simulink model "LugL6sStEnCtrl"  (R2018b)
settings: Solver=FixedStepDiscrete  StartTime=0.0  StopTime=10.0  FixedStep=0.01  RelTol=1e-3
undefined symbols (not defined in the file or in its folder): data, ThdRwLtStBkReclnEn_Clear, ThdRwLtStBkReclnEn_Set, ThdRwLtStFwdBkwdEn_Clear, ThdRwLtStFwdBkwdEn_Set
libraries: simulink x1
settings Model: Creator=sn2xws  LastModifiedBy=sn2xws
settings Model: ModifiedHistory=|
  | 2024.6.19 V1.0.0 557 模式流程
  | 2024.8.15 lug模式靠背一起动
settings DataIOCC: SaveFormat=StructureWithTime
settings OptimizationCC: DefaultParameterBehavior=Inlined  EnhancedBackFolding=on  PassReuseOutputArgsAs=Individual arguments  ZeroExternalMemoryAtStartup=off  ZeroInternalMemoryAtStartup=off  OptimizeBlockOrder=speed  DifferentSizesBufferReuse=on  OptimizationCustomize=off
settings DebuggingCC: ParameterTunabilityLossMsg=error
settings SFSimCC: MATLABDynamicMemAlloc=off
settings RTWCC: SystemTargetFile=autosar.tlc  GenCodeOnly=on  TemplateMakefile=ert_default_tmf  Description=AUTOSAR  GenerateReport=on  IncludeHyperlinkInReport=on  LaunchReport=on  GenerateTraceInfo=on  GenerateTraceReport=on  GenerateTraceReportSl=on  GenerateTraceReportSf=on  GenerateTraceReportEml=on
settings CodeAppCC: ForceParamTrailComments=on  IgnoreCustomStorageClasses=off  OperatorAnnotations=on  SimulinkDataObjDesc=on  SFDataObjDesc=on  InsertBlockDesc=on
settings STFCustomTargetCC: TargetLangStandard=C99 (ISO)  MultiwordLength=256  ParMdlRefBuildCompliant=on  CompOptLevelCompliant=on  IncludeMdlTerminateFcn=off  CombineOutputUpdateFcns=on  SuppressErrorStatus=on  ERTCustomFileBanners=on  SupportNonFinite=off  SupportComplex=off  SupportContinuousTime=off  SupportNonInlinedSFcns=off  RemoveResetFunc=on  MATLABClassNameForMDSCustomization=Simulink.SoftwareTarget.ERTCustomization  AutosarCompliant=on  UseToolchainInfoCompliant=on  LookupTableObjectStructAxisOrder=2,1,3,4,...  LUTObjectStructOrderEvenSpacing=Size,Table,Breakpoints  SystemTargetFile=autosar.tlc
settings ERTTargetCC: TargetLangStandard=C99 (ISO)  ConcurrentExecutionCompliant=off  IncludeMdlTerminateFcn=off  SuppressErrorStatus=on  SupportNonFinite=off  SupportComplex=off  ModelStepFunctionPrototypeControlCompliant=off  CPPClassGenCompliant=off  AutosarCompliant=on  LookupTableObjectStructAxisOrder=2,1,3,4,...  LUTObjectStructOrderEvenSpacing=Size,Table,Breakpoints  InlinedParameterPlacement=NonHierarchical  ERTCustomFileTemplate=example_file_process.tlc  ERTFilePackagingFormat=Compact

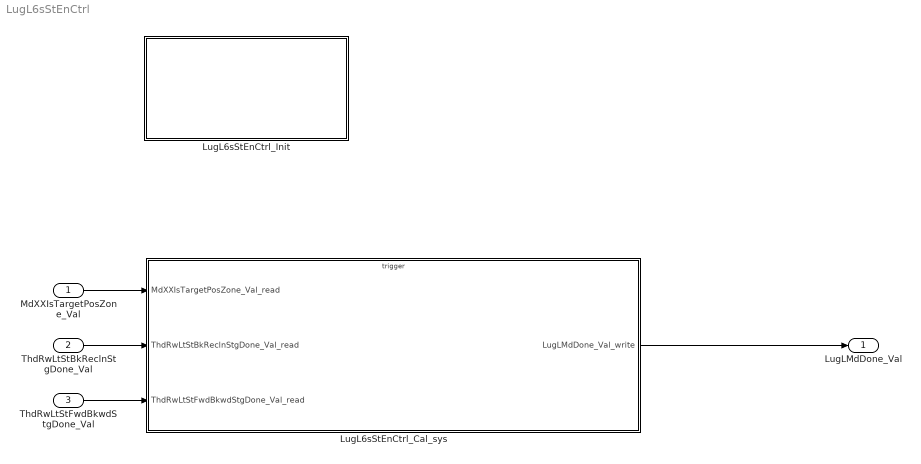
== system LugL6sStEnCtrl ==
  MdXXIsTargetPosZone_Val : Inport  OutDataTypeStr=uint32  PortDimensions=1
  ThdRwLtStBkReclnStgDone_Val : Inport  Port=2  OutDataTypeStr=boolean  PortDimensions=1
  ThdRwLtStFwdBkwdStgDone_Val : Inport  Port=3  OutDataTypeStr=boolean  PortDimensions=1
  LugL6sStEnCtrl_Cal_sys : Subsystem
  LugL6sStEnCtrl_Init : Subsystem
  LugLMdDone_Val : Outport  OutDataTypeStr=uint8  PortDimensions=1
  wires:
  MdXXIsTargetPosZone_Val/1 -> LugL6sStEnCtrl_Cal_sys/1(MdXXIsTargetPosZone_Val_read)
  ThdRwLtStBkReclnStgDone_Val/1 -> LugL6sStEnCtrl_Cal_sys/2(ThdRwLtStBkReclnStgDone_Val_read)
  ThdRwLtStFwdBkwdStgDone_Val/1 -> LugL6sStEnCtrl_Cal_sys/3(ThdRwLtStFwdBkwdStgDone_Val_read)
  LugL6sStEnCtrl_Cal_sys/1(LugLMdDone_Val_write) -> LugLMdDone_Val/1

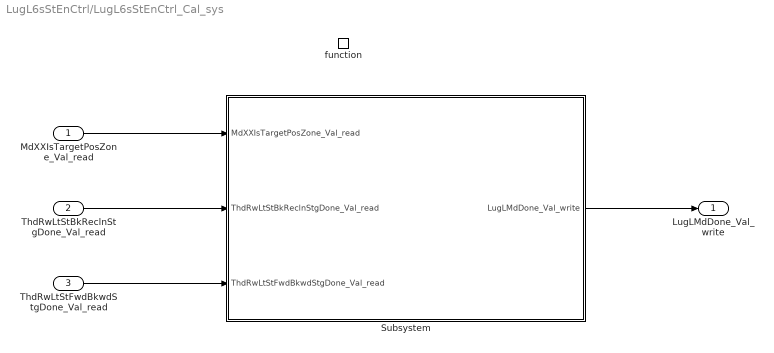
== system LugL6sStEnCtrl/LugL6sStEnCtrl_Cal_sys ==
  MdXXIsTargetPosZone_Val_read : Inport
  ThdRwLtStBkReclnStgDone_Val_read : Inport  Port=2
  ThdRwLtStFwdBkwdStgDone_Val_read : Inport  Port=3
  function : TriggerPort  TriggerType=function-call  IsSimulinkFunction=on  FunctionName=LugL6sStEnCtrl_Cal  VariantControl=(inherit)
  Subsystem : Subsystem
  LugLMdDone_Val_write : Outport
      settings: EnsureOutportIsVirtual=on
  wires:
  MdXXIsTargetPosZone_Val_read/1 -> Subsystem/1(MdXXIsTargetPosZone_Val_read)
  ThdRwLtStBkReclnStgDone_Val_read/1 -> Subsystem/2(ThdRwLtStBkReclnStgDone_Val_read)
  ThdRwLtStFwdBkwdStgDone_Val_read/1 -> Subsystem/3(ThdRwLtStFwdBkwdStgDone_Val_read)
  Subsystem/1(LugLMdDone_Val_write) -> LugLMdDone_Val_write/1

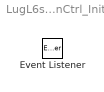
== system LugL6sStEnCtrl/LugL6sStEnCtrl_Init ==
  Event Listener : EventListener  EventName=reset

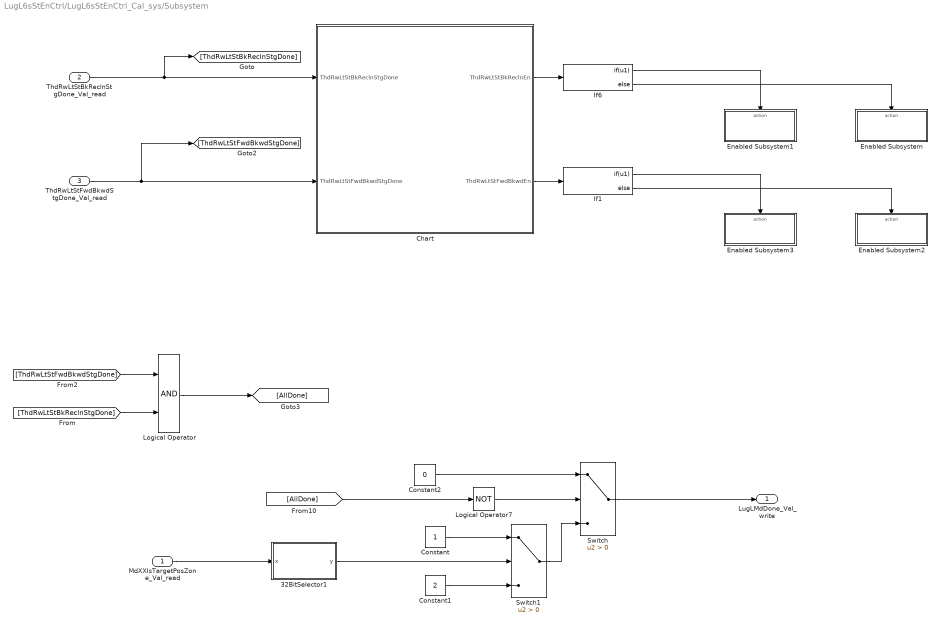
== system LugL6sStEnCtrl/LugL6sStEnCtrl_Cal_sys/Subsystem ==
  MdXXIsTargetPosZone_Val_read : Inport
  ThdRwLtStBkReclnStgDone_Val_read : Inport  Port=2
  ThdRwLtStFwdBkwdStgDone_Val_read : Inport  Port=3
  32BitSelector1 : Subsystem  mask(32 Bit Selector){BitNum=7}
      mask prompts: BitNum "Select Bit Number"
      mask help: Allows selection of a particular bit (0-31) out of a packed word up to 32 bits long. Output will be true if the bit number selected via the mask parameter is equal to one.
      mask TypeOptions BitNum: 0 | 1 | 2 | 3 | 4 | 5 | 6 | 7 | 8 | 9 | 10 | 11 | 12 | 13 | 14 | 15 | 16 | 17 | 18 | 19 | 20 | 21 | 22 | 23 | 24 | 25 | 26 | 27 | 28 | 29 | 30 | 31
      mask Display:
      | text(0.5, 0.8,'BIT','horizontalAlignment','center')
      | text(0.5, 0.5,'SELECTOR','horizontalAlignment','center')
      | text(0.5, 0.2,['-- Bit ',char(get_param(gcb,'BitNum')),' --'],'horizontalAlignment','center')
  Chart : Stateflow chart  TreatAsAtomicUnit=on
  Constant : Constant  OutDataTypeStr=uint8
  Constant1 : Constant  Value=2  OutDataTypeStr=uint8
  Constant2 : Constant  Value=0  OutDataTypeStr=uint8
  Enabled Subsystem : Subsystem  TreatAsAtomicUnit=on
  Enabled Subsystem1 : Subsystem  TreatAsAtomicUnit=on
  Enabled Subsystem2 : Subsystem  TreatAsAtomicUnit=on
  Enabled Subsystem3 : Subsystem  TreatAsAtomicUnit=on
  If1 : If  IfExpression=u1
  If6 : If  IfExpression=u1
  Logical Operator : Logic  AllPortsSameDT=off  OutDataTypeStr=boolean
  Logical Operator7 : Logic  Operator=NOT  AllPortsSameDT=off  OutDataTypeStr=boolean
  Switch : Switch  Criteria=u2 > Threshold
  Switch1 : Switch  Criteria=u2 > Threshold
  LugLMdDone_Val_write : Outport
      settings: EnsureOutportIsVirtual=on
  wires:
  Switch/1 -> LugLMdDone_Val_write/1
  Constant1/1 -> Switch1/3
  MdXXIsTargetPosZone_Val_read/1 -> 32BitSelector1/1(x)
  Switch1/1 -> Switch/3
  Logical Operator7/1 -> Switch/2
  Constant2/1 -> Switch/1
  Constant/1 -> Switch1/1
  [AllDone] -> Logical Operator7/1
  32BitSelector1/1(y) -> Switch1/2
  [ThdRwLtStBkReclnStgDone] -> Logical Operator/2
  Logical Operator/1 -> [AllDone]
  [ThdRwLtStFwdBkwdStgDone] -> Logical Operator/1
  ThdRwLtStBkReclnStgDone_Val_read/1 -> [ThdRwLtStBkReclnStgDone], Chart/1(ThdRwLtStBkReclnStgDone)
  ThdRwLtStFwdBkwdStgDone_Val_read/1 -> [ThdRwLtStFwdBkwdStgDone], Chart/2(ThdRwLtStFwdBkwdStgDone)
  If6/2 -> Enabled Subsystem/Action
  Chart/1(ThdRwLtStBkReclnEn) -> If6/1
  If6/1 -> Enabled Subsystem1/Action
  If1/1 -> Enabled Subsystem3/Action
  Chart/2(ThdRwLtStFwdBkwdEn) -> If1/1
  If1/2 -> Enabled Subsystem2/Action

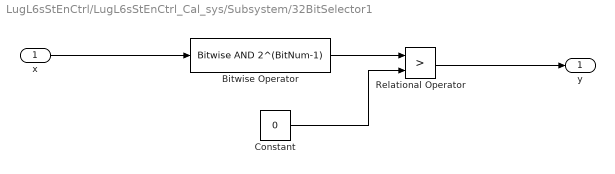
== system LugL6sStEnCtrl/LugL6sStEnCtrl_Cal_sys/Subsystem/32BitSelector1 ==
  x : Inport
  Bitwise Operator : simulink/Logic and Bit Operations/Bitwise Operator  logicop=AND  UseBitMask=on  BitMask=2^(BitNum-1)  BitMaskRealWorld=Stored Integer
  Constant : Constant  Value=0  OutDataTypeStr=uint32
  Relational Operator : RelationalOperator  Operator=>  OutDataTypeStr=boolean  RndMeth=Simplest
  y : Outport
  wires:
  Relational Operator/1 -> y/1
  Constant/1 -> Relational Operator/2
  x/1 -> Bitwise Operator/1
  Bitwise Operator/1 -> Relational Operator/1

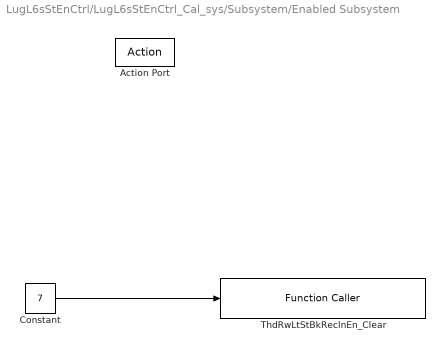
== system LugL6sStEnCtrl/LugL6sStEnCtrl_Cal_sys/Subsystem/Enabled Subsystem ==
  Action Port : ActionPort  ActionType=else
  Constant : Constant  Value=7  OutDataTypeStr=uint8
  ThdRwLtStBkReclnEn_Clear : FunctionCaller  FunctionPrototype=ThdRwLtStBkReclnEn_Clear(data)  InputArgumentSpecifications=uint8(1)
  wires:
  Constant/1 -> ThdRwLtStBkReclnEn_Clear/1

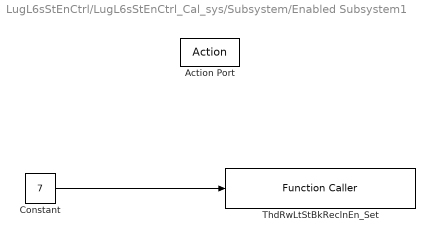
== system LugL6sStEnCtrl/LugL6sStEnCtrl_Cal_sys/Subsystem/Enabled Subsystem1 ==
  Action Port : ActionPort  ActionType=then
  Constant : Constant  Value=7  OutDataTypeStr=uint8
  ThdRwLtStBkReclnEn_Set : FunctionCaller  FunctionPrototype=ThdRwLtStBkReclnEn_Set(data)  InputArgumentSpecifications=uint8(1)
  wires:
  Constant/1 -> ThdRwLtStBkReclnEn_Set/1

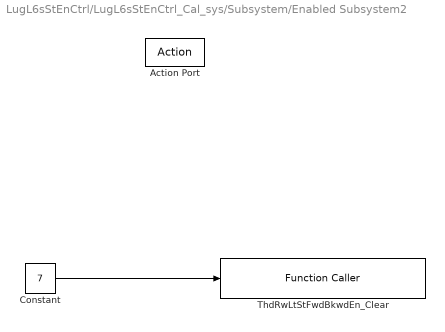
== system LugL6sStEnCtrl/LugL6sStEnCtrl_Cal_sys/Subsystem/Enabled Subsystem2 ==
  Action Port : ActionPort  ActionType=else
  Constant : Constant  Value=7  OutDataTypeStr=uint8
  ThdRwLtStFwdBkwdEn_Clear : FunctionCaller  FunctionPrototype=ThdRwLtStFwdBkwdEn_Clear(data)  InputArgumentSpecifications=uint8(1)
  wires:
  Constant/1 -> ThdRwLtStFwdBkwdEn_Clear/1

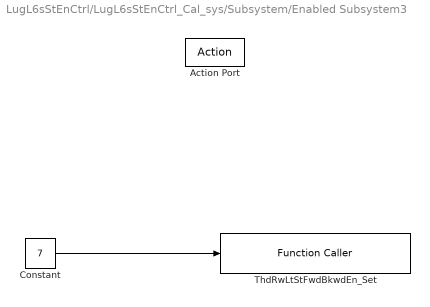
== system LugL6sStEnCtrl/LugL6sStEnCtrl_Cal_sys/Subsystem/Enabled Subsystem3 ==
  Action Port : ActionPort  ActionType=then
  Constant : Constant  Value=7  OutDataTypeStr=uint8
  ThdRwLtStFwdBkwdEn_Set : FunctionCaller  FunctionPrototype=ThdRwLtStFwdBkwdEn_Set(data)  InputArgumentSpecifications=uint8(1)
  wires:
  Constant/1 -> ThdRwLtStFwdBkwdEn_Set/1

== stateflow chart LugL6sStEnCtrl/LugL6sStEnCtrl_Cal_sys/Subsystem/Chart ==
  (default) -> (junction 9) : {
      | ThdRwLtStBkReclnEn = 0;
      | ThdRwLtStFwdBkwdEn = 0;
      | }
  (junction 9) -> (junction 49) [order 1] : [ThdRwLtStBkReclnStgDone]
  (junction 9) -> (junction 53) [order 2] : {
      | ThdRwLtStBkReclnEn=1;
      | }
  (junction 49) -> (junction 51)
  (junction 51) -> (junction 53)
  (junction 53) -> (junction 60)
  (junction 60) -> (junction 62) [order 1] : [ThdRwLtStFwdBkwdStgDone]
  (junction 60) -> (junction 66) [order 2] : {
      | ThdRwLtStFwdBkwdEn=1;
      | }
  (junction 62) -> (junction 64)
  (junction 64) -> (junction 66)
  data: ThdRwLtStBkReclnStgDone input boolean; ThdRwLtStFwdBkwdStgDone input boolean; ThdRwLtStBkReclnEn output boolean; ThdRwLtStFwdBkwdEn output boolean
